simulink model "simulink_model"  (R2025a)
settings: Solver=ode4  StartTime=0.0  StopTime=30  FixedStep=0.01  RelTol=1e-3
settings Model: Creator=User  LastModifiedBy=User

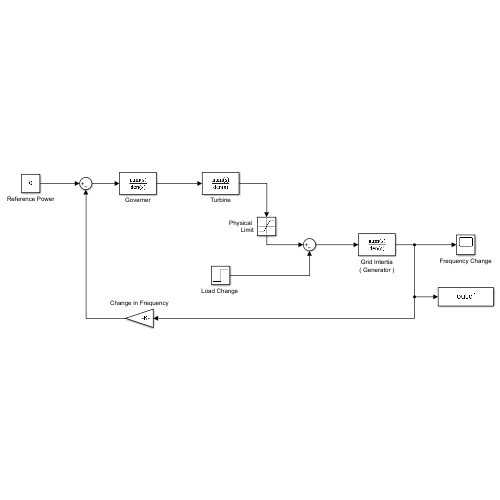
[thumbnail: Simulink's stored preview of the top-level diagram]
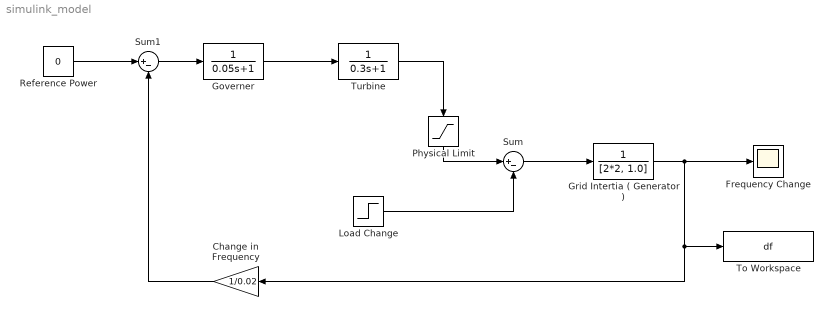
== system simulink_model ==
  Change in Frequency : Gain  Gain=1/0.02
  Frequency Change : Scope
      settings: ActiveDisplayYMinimum=-0.0045647831718082284  ActiveDisplayYMaximum=0.00062336521239743879
  Governer : TransferFcn  Denominator=[0.05 1]
  Grid Intertia ( Generator ) : TransferFcn  Denominator=[2*2, 1.0]
  "Load Change " : Step  Time=10  After=0.08  SampleTime=0
  Physical Limit : Saturate  UpperLimit=0.15  LowerLimit=0
  Reference Power : Constant  Value=0
  Sum : Sum  Inputs=|+-
  Sum1 : Sum  Inputs=|+-
  To Workspace : ToWorkspace  VariableName=df  SampleTime=-1
  Turbine : TransferFcn  Denominator=[0.3 1]
  wires:
  Governer/1 -> Turbine/1
  Turbine/1 -> Physical Limit/1
  "Load Change "/1 -> Sum/2
  Sum/1 -> Grid Intertia ( Generator )/1
  Grid Intertia ( Generator )/1 -> Change in Frequency/1, To Workspace/1, Frequency Change/1
  Sum1/1 -> Governer/1
  Change in Frequency/1 -> Sum1/2
  Physical Limit/1 -> Sum/1
  Reference Power/1 -> Sum1/1
